simulink model "BoatSim"  (R2018a)
settings: Solver=ode45  StartTime=0.0  StopTime=50  RelTol=1e-3  EnableMultiTasking=on
undefined symbols (not defined in the file or in its folder): Dr, dSamplingPeriod, Du, Dv, IoM, Mass, OM, rg, sigbuilder_block
libraries: simulink x1
settings Model: Creator=hamada  LastModifiedBy=shuhei
settings DataIOCC: LimitDataPoints=on  SaveFormat=Array
settings OptimizationCC: LifeSpan=inf
settings DebuggingCC: SFUnexpectedBacktrackingDiag=warning  SFNoUnconditionalDefaultTransitionDiag=warning  SFExecutionAtInitializationDiag=none
settings HardwareCC: ProdBitPerPointer=32  ProdBitPerSizeT=32  ProdBitPerPtrDiffT=32  ProdLargestAtomicFloat=None  ProdIntDivRoundTo=Undefined  ProdEndianess=Unspecified  ProdWordSize=32  ProdHWDeviceType=32-bit Generic
settings ModelReferenceCC: PropagateSignalLabelsOutOfModel=off
settings CodeAppCC: StateflowObjectComments=on
settings GRTTargetCC: TargetLangStandard=C89/C90 (ANSI)  GeneratePreprocessorConditionals=Disable all
settings ConfigComp: CovMetricSettings=dw  CovHtmlReporting=on  CovSaveCumulativeToWorkspaceVar=on  CovSaveSingleToWorkspaceVar=on  CovExternalEMLEnable=off

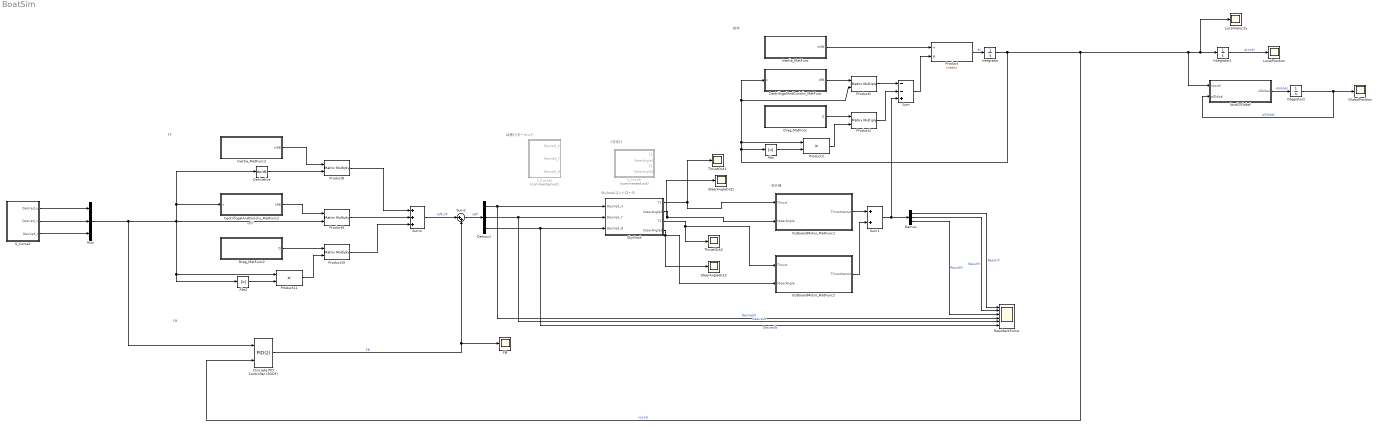
== system BoatSim ==
  note: 船外機
  note: 船体
  note: S字走行
  note: 目標力/モーメント
  note: Skyhookコントローラ
  note: FF
  note: FB
  Abs : Abs
  Abs2 : Abs
  CentrifugalAndCoriolis_MatFunc : MATLAB Function  TreatAsAtomicUnit=on
  CentrifugalAndCoriolis_MatFunc2 : MATLAB Function  TreatAsAtomicUnit=on
  Demux : Demux  Outputs=3
  Demux1 : Demux  Outputs=3
  Derivative : Derivative
  Discrete PID Controller (2DOF) : simulink/Continuous/PID Controller (2DOF)  Controller=PID  TimeDomain=Discrete-time  SampleTime=-1  IntegratorMethod=Forward Euler  FilterMethod=Forward Euler  Form=Parallel  UseFilter=on  ControllerParametersSource=internal  P=1000  I=0  D=0  N=100  b=1  c=1  InitialConditionSource=internal  InitialConditionForIntegrator=0  InitialConditionForFilter=0  ExternalReset=none  ZeroCross=off  LimitOutput=off  UpperSaturationLimit=inf  LowerSaturationLimit=-inf  LinearizeAsGain=off  AntiWindupMode=none  Kb=1  TrackingMode=off  Kt=1  PParamMin=[]  PParamMax=[]  IParamMin=[]  IParamMax=[]  DParamMin=[]  DParamMax=[]  NParamMin=[]  NParamMax=[]  bParamMin=[]  bParamMax=[]  cParamMin=[]  cParamMax=[]  KbParamMin=[]  KbParamMax=[]  KtParamMin=[]  KtParamMax=[]  POutMin=[]  POutMax=[]  IOutMin=[]  IOutMax=[]  DOutMin=[]  DOutMax=[]  NOutMin=[]  NOutMax=[]  bOutMin=[]  bOutMax=[]  cOutMin=[]  cOutMax=[]  KbOutMin=[]  KbOutMax=[]  KtOutMin=[]  KtOutMax=[]  IntegratorOutMin=[]  IntegratorOutMax=[]  FilterOutMin=[]  FilterOutMax=[]  SumOutMin=[]  SumOutMax=[]  Sum1OutMin=[]  Sum1OutMax=[]  Sum2OutMin=[]  Sum2OutMax=[]  Sum3OutMin=[]  Sum3OutMax=[]  SumI1OutMin=[]  SumI1OutMax=[]  SumI2OutMin=[]  SumI2OutMax=[]  SumI3OutMin=[]  SumI3OutMax=[]  SumDOutMin=[]  SumDOutMax=[]  SaturationOutMin=[]  SaturationOutMax=[]  IntegratorContinuousStateAttributes=''  IntegratorStateMustResolveToSignalObject=off  IntegratorRTWStateStorageClass=Auto  FilterContinuousStateAttributes=''  FilterStateMustResolveToSignalObject=off  FilterRTWStateStorageClass=Auto  DifferentiatorICPrevScaledInput=0  DifferentiatorOutMin=[]  DifferentiatorOutMax=[]  FilterDiffOutCoefMin=[]  FilterDiffOutCoefMax=[]  SumDenOutMin=[]  SumDenOutMax=[]  SumNumOutMin=[]  SumNumOutMax=[]  ReciprocalOutMin=[]  ReciprocalOutMax=[]  DivideOutMin=[]  DivideOutMax=[]  TunerSelectOption=Transfer Function Based (PID Tuner App)
  Drag_MatFunc : MATLAB Function  TreatAsAtomicUnit=on
  Drag_MatFunc2 : MATLAB Function  TreatAsAtomicUnit=on
  FB : Scope
  GlobalPosition : Scope
  Inertia_MatFunc : MATLAB Function  TreatAsAtomicUnit=on
  Inertia_MatFunc2 : MATLAB Function  TreatAsAtomicUnit=on
  Integrator : Integrator
  Integrator1 : Integrator
  Integrator2 : Integrator
  LocalPosition : Scope
  "LocalVelocity " : Scope
  Mux : Mux  Inputs=3
  OutboardMotor_MatFunc1 : MATLAB Function  TreatAsAtomicUnit=on
  OutboardMotor_MatFunc2 : MATLAB Function  TreatAsAtomicUnit=on
  Product : Product  Inputs=/*  Multiplication=Matrix(*)
  Product{1..2,8..10} (5 alike) : Product  Multiplication=Matrix(*)
  Product11 : Product
  Product3 : Product
  ResultantForce : Scope  NumInputPorts=6
  S_Curve : Subsystem  Commented=on
  S_Curve1 : Subsystem  Tag=STV Subsys  Commented=on  LoadFcn=sigbuilder_block('load');  StartFcn=sigbuilder_block('start');  StopFcn=sigbuilder_block('stop');  ClipboardFcn=sigbuilder_block('clipboard');  mask(Sigbuilder block){tuvar=[0:10]}
      mask help: Simulink:masks:SigbuilderBlock_MD
      mask init:
      | if ~strcmp(get_param(bdroot(gcbh),'SimulationStatus'),'stopped') tuvar = sigbuilder_block('maskInit'); end
      settings: CopyFcn=sigbuilder_block('copy');  DeleteFcn=sigbuilder_block('delete');  ModelCloseFcn=sigbuilder_block('modelClose');  PreSaveFcn=sigbuilder_block('preSave');  PauseFcn=sigbuilder_block('pause');  ContinueFcn=sigbuilder_block('continue');  NameChangeFcn=sigbuilder_block('namechange');  OpenFcn=sigbuilder_block('open',[674 298 550 400 ]);  CloseFcn=sigbuilder_block('close');
      mask Display: plot(0, 0, 100, 100,[2, 2, 32, 32, 2], [68, 8, 8, 68, 68],[32, 2], [38, 38], [32, 19, 2],[53, 60, 44], [32, 17, 17, 2],[16, 16, 31, 31]);txt = getActiveGroup(gcbh);text(2, 100, txt,'verticalAlignment', 'top');
  S_Curve2 : Subsystem  Tag=STV Subsys  LoadFcn=sigbuilder_block('load',[0 0 942 582 ]);  StartFcn=sigbuilder_block('start');  StopFcn=sigbuilder_block('stop');  ClipboardFcn=sigbuilder_block('clipboard');  mask(Sigbuilder block){tuvar=[0:10]}
      mask help: Simulink:masks:SigbuilderBlock_MD
      mask init:
      | if ~strcmp(get_param(bdroot(gcbh),'SimulationStatus'),'stopped') tuvar = sigbuilder_block('maskInit'); end
      settings: CopyFcn=sigbuilder_block('copy');  DeleteFcn=sigbuilder_block('delete');  ModelCloseFcn=sigbuilder_block('modelClose');  PreSaveFcn=sigbuilder_block('preSave');  PauseFcn=sigbuilder_block('pause');  ContinueFcn=sigbuilder_block('continue');  NameChangeFcn=sigbuilder_block('namechange');  OpenFcn=sigbuilder_block('open',[674 298 550 400 ]);  CloseFcn=sigbuilder_block('close');
      mask Display: plot(0, 0, 100, 100,[2, 2, 32, 32, 2], [68, 8, 8, 68, 68],[32, 2], [38, 38], [32, 19, 2],[53, 60, 44], [32, 17, 17, 2],[16, 16, 31, 31]);txt = getActiveGroup(gcbh);text(2, 100, txt,'verticalAlignment', 'top');
  SkyHook : Subsystem
  SteerAngleOut1 : Scope
  SteerAngleOut2 : Scope
  Sum : Sum  Inputs=--+
  Sum1 : Sum
  Sum2 : Sum  Inputs=|++
  Sum4 : Sum  Inputs=+++
  ThrustOut1 : Scope
  ThrustOut2 : Scope
  local2Global : MATLAB Function  TreatAsAtomicUnit=on
  wires:
  Inertia_MatFunc/1(mRB) -> Product/1
  Product/1 -> Integrator/1  "dv"
  Integrator/1 -> Discrete PID Controller (2DOF)/2, local2Global/1(vLocal), "LocalVelocity "/1, Integrator1/1, Abs/1, Product3/1, CentrifugalAndCoriolis_MatFunc/1(v), Product2/2  "vLocal"
  Integrator1/1 -> LocalPosition/1  "pLocal"
  CentrifugalAndCoriolis_MatFunc/1(cRB) -> Product2/1
  Product2/1 -> Sum/1
  Drag_MatFunc/1(D) -> Product1/1
  Sum/1 -> Product/2
  local2Global/1(vGlobal) -> Integrator2/1  "vGlobal"
  Integrator2/1 -> local2Global/2(pGlobal), GlobalPosition/1  "pGlobal"
  Sum1/1 -> Demux/1, Sum/3
  OutboardMotor_MatFunc1/1(ThrustVector) -> Sum1/1
  OutboardMotor_MatFunc2/1(ThrustVector) -> Sum1/2
  SkyHook/4(SteerAngle2) -> SteerAngleOut2/1, OutboardMotor_MatFunc2/2(SteerAngle)
  SkyHook/3(T2) -> OutboardMotor_MatFunc2/1(Thrust), ThrustOut2/1
  SkyHook/1(T1) -> OutboardMotor_MatFunc1/1(Thrust), ThrustOut1/1
  Demux/1 -> ResultantForce/1  "ResultX"
  Demux/2 -> ResultantForce/2  "ResultY"
  Demux/3 -> ResultantForce/3  "ResultN"
  Product1/1 -> Sum/2
  Product3/1 -> Product1/2
  Abs/1 -> Product3/2
  S_Curve2/1(Desired_u) -> Mux/1
  S_Curve2/2(Desired_v) -> Mux/2
  S_Curve2/3(Desired_r) -> Mux/3
  Inertia_MatFunc2/1(mRB) -> Product8/1
  Derivative/1 -> Product8/2
  CentrifugalAndCoriolis_MatFunc2/1(cRB) -> Product9/1
  Abs2/1 -> Product11/2
  Mux/1 -> Discrete PID Controller (2DOF)/1, Product11/1, Abs2/1, Derivative/1, CentrifugalAndCoriolis_MatFunc2/1(v), Product9/2  "refV"
  Product11/1 -> Product10/2
  Drag_MatFunc2/1(D) -> Product10/1
  Product8/1 -> Sum4/1
  Product9/1 -> Sum4/2
  Product10/1 -> Sum4/3
  Demux1/1 -> ResultantForce/4, SkyHook/1(Desired_X)  "DesiredX"
  Demux1/3 -> ResultantForce/6, SkyHook/3(Desired_N)  "DesiredN"
  Sum4/1 -> Sum2/1  "refF_FF"
  Demux1/2 -> ResultantForce/5, SkyHook/2(Desired_Y)  "DesiredY"
  SkyHook/2(SteerAngle1) -> SteerAngleOut1/1, OutboardMotor_MatFunc1/2(SteerAngle)
  Sum2/1 -> Demux1/1  "refF"
  Discrete PID Controller (2DOF)/1 -> FB/1, Sum2/2  "FB"

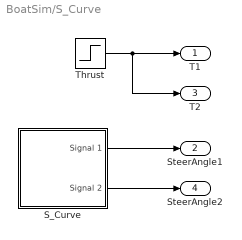
== system BoatSim/S_Curve ==
  S_Curve : Subsystem  Tag=STV Subsys  LoadFcn=sigbuilder_block('load');  StartFcn=sigbuilder_block('start');  StopFcn=sigbuilder_block('stop');  ClipboardFcn=sigbuilder_block('clipboard');  mask(Sigbuilder block){tuvar=[0:10]}
      mask help: Simulink:masks:SigbuilderBlock_MD
      mask init:
      | if ~strcmp(get_param(bdroot(gcbh),'SimulationStatus'),'stopped') tuvar = sigbuilder_block('maskInit'); end
      settings: CopyFcn=sigbuilder_block('copy');  DeleteFcn=sigbuilder_block('delete');  ModelCloseFcn=sigbuilder_block('modelClose');  PreSaveFcn=sigbuilder_block('preSave');  PauseFcn=sigbuilder_block('pause');  ContinueFcn=sigbuilder_block('continue');  NameChangeFcn=sigbuilder_block('namechange');  OpenFcn=sigbuilder_block('open',[437.6 199.2 550.4 400 ]);  CloseFcn=sigbuilder_block('close');
      mask Display: plot(0, 0, 100, 100,[2, 2, 32, 32, 2], [68, 8, 8, 68, 68],[32, 2], [38, 38], [32, 19, 2],[53, 60, 44], [32, 17, 17, 2],[16, 16, 31, 31]);txt = getActiveGroup(gcbh);text(2, 100, txt,'verticalAlignment', 'top');
  Thrust : Step  After=[1000;0;]  SampleTime=0
  T1 : Outport
  SteerAngle1 : Outport  Port=2
  T2 : Outport  Port=3
  SteerAngle2 : Outport  Port=4
  wires:
  Thrust/1 -> T2/1, T1/1
  S_Curve/1(Signal 1) -> SteerAngle1/1
  S_Curve/2(Signal 2) -> SteerAngle2/1

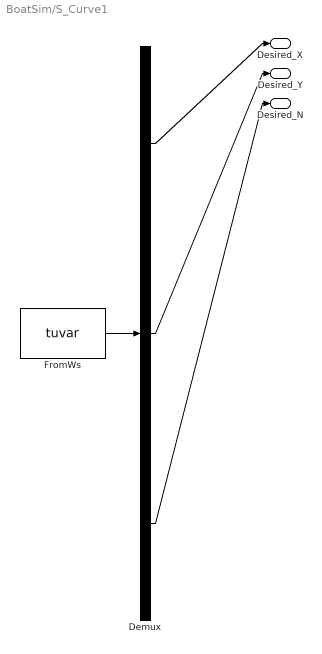
== system BoatSim/S_Curve1 ==
  Demux : Demux  Tag=STV Demux  Outputs=3
  FromWs : FromWorkspace  Tag=STV FromWs  VariableName=tuvar  SampleTime=0
      SigBuilderData=|
      | common.afterFinalStr = 'Extrapolate'
      | common.sampleTime = 0
      | dataSet.timeRange = [0 50]
      | dataSet.name = 'Group 1'
      | sbobj.Groups.Name = 'Group 1'
      | sbobj.Groups.Signals(1).Name = 'Desired_X'
      | sbobj.Groups.Signals(1).XData = [0 16 17 35 50]
      | sbobj.Groups.Signals(1).YData = [0 0 0 0 0]
      | sbobj.Groups.Signals(2).Name = 'Desired_Y'
      | sbobj.Groups.Signals(2).XData = [0 10 20 20 35 35 50]
      | sbobj.Groups.Signals(2).YData = [0 0 0 -0.123 -0.123 0 0]
      | sbobj.Groups.Signals(3).Name = 'Desired_N'
      | sbobj.Groups.Signals(3).XData = [0 28 30 50]
      | sbobj.Groups.Signals(3).YData = [0 0 0 0]
      | sbobj.Groups.TimeRange = [0 50]
  Desired_X : Outport  Tag=STV Outport
  Desired_Y : Outport  Tag=STV Outport  Port=2
  Desired_N : Outport  Tag=STV Outport  Port=3
  wires:
  FromWs/1 -> Demux/1
  Demux/1 -> Desired_X/1
  Demux/2 -> Desired_Y/1
  Demux/3 -> Desired_N/1

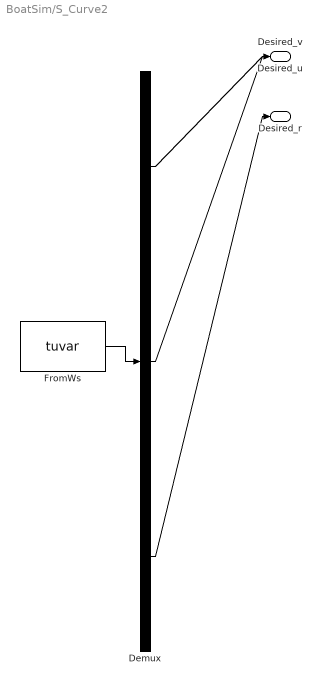
== system BoatSim/S_Curve2 ==
  Demux : Demux  Tag=STV Demux  Outputs=3
  FromWs : FromWorkspace  Tag=STV FromWs  VariableName=tuvar  SampleTime=0
      SigBuilderData=|
      | common.afterFinalStr = 'Extrapolate'
      | common.sampleTime = 0
      | dataSet(1).timeRange = [0 50]
      | dataSet(1).name = 'Group 2'
      | dataSet(2).timeRange = [0 50]
      | dataSet(2).name = 'Group 1'
      | sbobj.Groups(1).Name = 'Group 2'
      | sbobj.Groups(1).Signals(1).Name = 'Desired_u'
      | sbobj.Groups(1).Signals(1).XData = [0 5 10 15 50]
      | sbobj.Groups(1).Signals(1).YData = [0 1 1 0 0]
      | sbobj.Groups(1).Signals(2).Name = 'Desired_v'
      | sbobj.Groups(1).Signals(2).XData = [0 20 25 30 35 50]
      | sbobj.Groups(1).Signals(2).YData = [0 0 0.1 0.1 0 0]
      | sbobj.Groups(1).Signals(3).Name = 'Desired_r'
      | sbobj.Groups(1).Signals(3).XData = [0 28 30 50]
      | sbobj.Groups(1).Signals(3).YData = [0 0.48 0 0]
      | sbobj.Groups(1).TimeRange = [0 50]
      | sbobj.Groups(2).Name = 'Group 1'
      | sbobj.Groups(2).Signals(1).Name = 'Desired_u'
      | sbobj.Groups(2).Signals(1).XData = [0 1.05263157895 2.10526315789 3.15789473684 4.21052631579 5.26315789474 6.31578947368 7.36842105263 8.42105263158 9.47368421053 10.5263157895 11.5789473684 12.6315789474 13.6842105263 14.7368421053 15.7894736842 16.8421052632 17.8947368421 18.9473684211 20 21.0526315789 22.1052631579 23.1578947368 24.2105263158 25.2631578947 26.3157894737 27.3684210526 28.4210526316 29.4736842105 30.5263157895 31.5789473684 32.6315789474 33.6842105263 34.7368421053 35.7894736842 36.8421052632 37.8947368421 38.9473684211 40 41.0526315789 42.1052631579 43.1578947368 44.2105263158 45.2631578947 46.3157894737 47.3684210526 48.4210526316 49.4736842105 50]
      | sbobj.Groups(2).Signals(1).YData = [0 0.162349734602 0.307106356345 0.418583239131 0.48470013297 0.498292246503 0.457886663328 0.367861955337 0.237973696519 0.0822972951404 -0.0822972951404 -0.237973696519 -0.367861955337 -0.457886663328 -0.498292246503 -0.48470013297 -0.418583239131 -0.307106356345 -0.162349734602 0 0.162349734602 0.307106356345 0.418583239131 0.48470013297 0.498292246503 0.457886663328 0.367861955337 0.237973696519 0.0822972951404 -0.0822972951404 -0.237973696519 -0.367861955337 -0.457886663328 -0.498292246503 -0.48470013297 -0.418583239131 -0.307106356345 -0.162349734602 0 0.162349734602 0.307106356345 0.418583239131 0.48470013297 0.498292246503 0.457886663328 0.367861955337 0.237973696519 0.0822972951404 -5.82016719913e-16]
      | sbobj.Groups(2).Signals(2).Name = 'Desired_v'
      | sbobj.Groups(2).Signals(2).XData = [0 50]
      | sbobj.Groups(2).Signals(2).YData = [0 0]
      | sbobj.Groups(2).Signals(3).Name = 'Desired_r'
      | sbobj.Groups(2).Signals(3).XData = [0 28 30 50]
      | sbobj.Groups(2).Signals(3).YData = [0 0.08 -0.14 0]
      | sbobj.Groups(2).TimeRange = [0 50]
  Desired_u : Outport  Tag=STV Outport
  Desired_v : Outport  Tag=STV Outport  Port=2
  Desired_r : Outport  Tag=STV Outport  Port=3
  wires:
  FromWs/1 -> Demux/1
  Demux/1 -> Desired_u/1
  Demux/2 -> Desired_v/1
  Demux/3 -> Desired_r/1

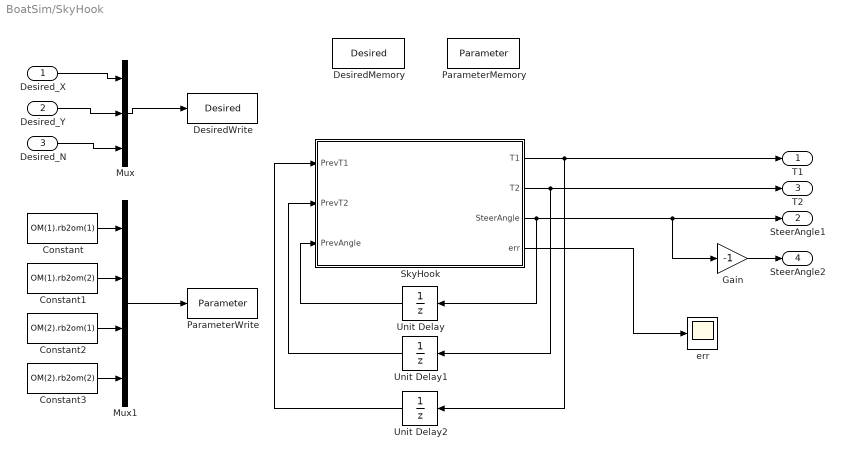
== system BoatSim/SkyHook ==
  Desired_X : Inport
  Desired_Y : Inport  Port=2
  Desired_N : Inport  Port=3
  Constant : Constant  Value=OM(1).rb2om(1)
  Constant1 : Constant  Value=OM(1).rb2om(2)
  Constant2 : Constant  Value=OM(2).rb2om(1)
  Constant3 : Constant  Value=OM(2).rb2om(2)
  DesiredMemory : DataStoreMemory  DataStoreName=Desired  ReadBeforeWriteMsg=warning  WriteAfterWriteMsg=warning  WriteAfterReadMsg=warning  InitialValue=[0;0;0;]  ShowAdditionalParam=off  OutDataTypeStr=double  Dimensions=3
  DesiredWrite : DataStoreWrite  DataStoreName=Desired
  Gain : Gain  Gain=-1
  Mux : Mux  Inputs=3
  Mux1 : Mux
  ParameterMemory : DataStoreMemory  DataStoreName=Parameter  ReadBeforeWriteMsg=warning  WriteAfterWriteMsg=warning  WriteAfterReadMsg=warning  InitialValue=[0;0;0;0;]  ShowAdditionalParam=off  OutDataTypeStr=double  Dimensions=4
  ParameterWrite : DataStoreWrite  DataStoreName=Parameter
  SkyHook : MATLAB Function  TreatAsAtomicUnit=on  SystemSampleTime=dSamplingPeriod
  Unit Delay : UnitDelay  SampleTime=-1
  Unit Delay1 : UnitDelay  SampleTime=-1
  Unit Delay2 : UnitDelay  SampleTime=-1
  "err " : Scope
  T1 : Outport
  SteerAngle1 : Outport  Port=2
  T2 : Outport  Port=3
  SteerAngle2 : Outport  Port=4
  wires:
  Mux/1 -> DesiredWrite/1
  Desired_X/1 -> Mux/1
  Desired_Y/1 -> Mux/2
  Desired_N/1 -> Mux/3
  Mux1/1 -> ParameterWrite/1
  Constant/1 -> Mux1/1
  Constant1/1 -> Mux1/2
  Constant2/1 -> Mux1/3
  Constant3/1 -> Mux1/4
  SkyHook/2(T2) -> Unit Delay1/1, T2/1
  SkyHook/3(SteerAngle) -> SteerAngle1/1, Gain/1, Unit Delay/1
  Gain/1 -> SteerAngle2/1
  SkyHook/4(err) -> "err "/1
  Unit Delay1/1 -> SkyHook/2(PrevT2)
  Unit Delay2/1 -> SkyHook/1(PrevT1)
  SkyHook/1(T1) -> Unit Delay2/1, T1/1
  Unit Delay/1 -> SkyHook/3(PrevAngle)

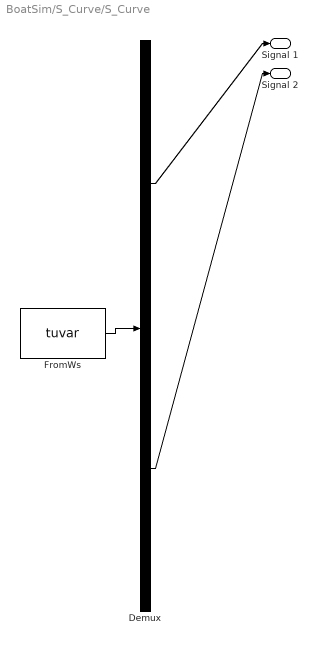
== system BoatSim/S_Curve/S_Curve ==
  Demux : Demux  Tag=STV Demux  Outputs=2
  FromWs : FromWorkspace  Tag=STV FromWs  VariableName=tuvar  SampleTime=0
      SigBuilderData=|
      | common.afterFinalStr = 'Extrapolate'
      | common.sampleTime = 0
      | dataSet.timeRange = [0 50]
      | dataSet.name = 'Group 1'
      | sbobj.Groups.Name = 'Group 1'
      | sbobj.Groups.Signals(1).Name = 'Signal 1'
      | sbobj.Groups.Signals(1).XData = [0 5 10 15 20 25 25 30 35 50]
      | sbobj.Groups.Signals(1).YData = [0 0 0.523598775598 0.523598775598 0 -0.523598775598 -0.52 -0.523598775598 0 0]
      | sbobj.Groups.Signals(2).Name = 'Signal 2'
      | sbobj.Groups.Signals(2).XData = [0 5 10 15 20 25 25 30 35 50]
      | sbobj.Groups.Signals(2).YData = [0 0 0.523598775598 0.523598775598 0 -0.523598775598 -0.52 -0.523598775598 0 0]
      | sbobj.Groups.TimeRange = [0 50]
  Signal 1 : Outport  Tag=STV Outport
  Signal 2 : Outport  Tag=STV Outport  Port=2
  wires:
  FromWs/1 -> Demux/1
  Demux/1 -> Signal 1/1
  Demux/2 -> Signal 2/1

== matlab function BoatSim/CentrifugalAndCoriolis_MatFunc ==
  data: v input size=3; Mass parameter size=1; rg parameter size=2; cRB output size=3,3
function cRB = CentrifugalAndCoriolis_MatFunc( v, Mass, rg )
    cRB = CentrifugalAndCoriolis( Mass, rg, v );
end

== matlab function BoatSim/Inertia_MatFunc ==
  data: Mass parameter size=1; mRB output size=3,3; IoM parameter size=1; rg parameter size=2
function mRB = Inertia_MatFunc( Mass, IoM, rg )
    mRB = Inertia( Mass, IoM, rg );
end

== matlab function BoatSim/Drag_MatFunc ==
  data: Du parameter size=1; Dv parameter size=1; D output size=3,3; Dr parameter size=1
function D = Drag_MatFunc( Du, Dv, Dr )
    D = Drag( Du, Dv, Dr );
end

== matlab function BoatSim/local2Global ==
  data: vLocal input size=3; vGlobal output size=3; pGlobal input size=3
function vGlobal = local2global_MatFunc( vLocal, pGlobal )
    vGlobal = local2global( vLocal, pGlobal );
end

== matlab function BoatSim/OutboardMotor_MatFunc1 ==
  data: Thrust input size=2; ThrustVector output size=3; SteerAngle input size=1; rg parameter size=2; OM parameter
function ThrustVector = OutboardMotor_MatFunc( Thrust, SteerAngle, rg, OM )
    ThrustVector = OutboardMotor( Thrust, SteerAngle, rg, OM(1).rb2om );
end

== matlab function BoatSim/OutboardMotor_MatFunc2 ==
  data: Thrust input size=2; ThrustVector output size=3; SteerAngle input size=1; rg parameter size=2; OM parameter
function ThrustVector = OutboardMotor_MatFunc( Thrust, SteerAngle, rg, OM )
    ThrustVector = OutboardMotor( Thrust, SteerAngle, rg, OM(2).rb2om );
end

== matlab function BoatSim/SkyHook/SkyHook ==
  data: T1 output size=2; T2 output size=2; SteerAngle output size=1; Desired data_store_memory size=4; Parameter data_store_memory; err output; PrevT1 input; PrevT2 input; PrevAngle input
function [ T1, T2, SteerAngle, err]  = SkyHook_MatFunc(PrevT1,PrevT2,PrevAngle)
    % 初期値
    x_initial = [100,100,0.1];%[PrevT1(1);PrevT2(1);PrevAngle;];
    
    % 最適化の実行
    [x,err1] = fminsearch( @ObjectiveFunction, x_initial );
    
    % 初期値
    %x_initial = [PrevT1(1);PrevT2(1);0.1;];%PrevAngle;];
    
    % 最適化の実行
    %[x2,err2] = fminsearch( @ObjectiveFunction, x_initial );

    % 最適化により求めたスラスト/ステアリング角を出力
    T1 = [ x(1);0; ];
    T2 = [ x(2);0; ];
    SteerAngle = x(3);

    % 収束の確認
    global Desired;
    global Parameter;
    
    Desired_X = Desired(1); % 目標とするX方向にはたらく力
    Desired_Y = Desired(2); % 目標とするY方向にはたらく力
    Desired_N = Desired(3); % 目標とするヨー方向のモーメント

    OM1_rb2om_X = Parameter(1); % 船体重心から船外機1までのX方向距離
    OM1_rb2om_Y = Parameter(2); % 船体重心から船外機1までのY方向距離
    OM2_rb2om_X = Parameter(3); % 船体重心から船外機2までのX方向距離
    OM2_rb2om_Y = Parameter(4); % 船体重心から船外機2までのY方向距離
    
    X_T1 = T1(1) * cos( SteerAngle );
    Y_T1 = T1(1) * sin( SteerAngle );
    
    % 船外機2のスラスト
    X_T2 = T2(1) * cos( -SteerAngle );
    Y_T2 = T2(1) * sin( -SteerAngle );

    % X方向合力
    X = X_T1 + X_T2;
    % Y方向合力
    Y = Y_T1 + Y_T2;
    % モーメントの和
    N = ( OM1_rb2om_X * Y_T1 - OM1_rb2om_Y * X_T1 ) + ( OM2_rb2om_X * Y_T2 - OM2_rb2om_Y * X_T2 );

    err = [X;Desired_X;Y;Desired_Y;N; Desired_N;];
end

function ret = ObjectiveFunction( x0 )
    % 評価関数の重み付けのためのベースライン
    X0=1.;
    Y0=1.;
    N0=1.;
    T0=1e9;
    A0=1e9;
    
    global Desired;
    global Parameter;
    
    Desired_X = Desired(1); % 目標とするX方向にはたらく力
    Desired_Y = Desired(2); % 目標とするY方向にはたらく力
    Desired_N = Desired(3); % 目標とするヨー方向のモーメント

    OM1_rb2om_X = Parameter(1); % 船体重心から船外機1までのX方向距離
    OM1_rb2om_Y = Parameter(2); % 船体重心から船外機1までのY方向距離
    OM2_rb2om_X = Parameter(3); % 船体重心から船外機2までのX方向距離
    OM2_rb2om_Y = Parameter(4); % 船体重心から船外機2までのY方向距離
    
    % 最適化変数x0のリネーム
    T1 = x0(1);
    T2 = x0(2);
    SteerAngle = x0(3);

    % 船外機1のスラスト
    X_T1 = T1 * cos( SteerAngle );
    Y_T1 = T1 * sin( SteerAngle );
    
    % 船外機2のスラスト
    X_T2 = T2 * cos( -SteerAngle );
    Y_T2 = T2 * sin( -SteerAngle );

    % X方向合力
    X = X_T1 + X_T2;
    % Y方向合力
    Y = Y_T1 + Y_T2;
    % モーメントの和
    N = ( OM1_rb2om_X * Y_T1 - OM1_rb2om_Y * X_T1 ) + ( OM2_rb2om_X * Y_T2 - OM2_rb2om_Y * X_T2 );

    % 評価函数の値を返却
    ret = ( Desired_X - X )^2/(X0^2) + ( Desired_Y - Y )^2/(Y0^2) + ( Desired_N - N )^2/(N0^2) + T1^2/(T0^2) + T2^2/(T0^2) + SteerAngle^2/(A0^2);
end

== matlab function BoatSim/Inertia_MatFunc2 ==
  data: Mass parameter size=1; mRB output size=3,3; IoM parameter size=1; rg parameter size=2
function mRB = Inertia_MatFunc( Mass, IoM, rg )
    mRB = Inertia( Mass, IoM, rg );
end

== matlab function BoatSim/CentrifugalAndCoriolis_MatFunc2 ==
  data: v input size=3; Mass parameter size=1; rg parameter size=2; cRB output size=3,3
function cRB = CentrifugalAndCoriolis_MatFunc( v, Mass, rg )
    cRB = CentrifugalAndCoriolis( Mass, rg, v );
end

== matlab function BoatSim/Drag_MatFunc2 ==
  data: Du parameter size=1; Dv parameter size=1; D output size=3,3; Dr parameter size=1
function D = Drag_MatFunc( Du, Dv, Dr )
    D = Drag( Du, Dv, Dr );
end
